simulink model "windModel"  (R2024a)
settings: Solver=VariableStepAuto  StartTime=0.0  StopTime=30  RelTol=1e-3
undefined symbols (not defined in the file or in its folder): F, MIL, Moderate
libraries: aerolibwind2 x2
settings Model: Creator=franklinho  LastModifiedBy=franklinho

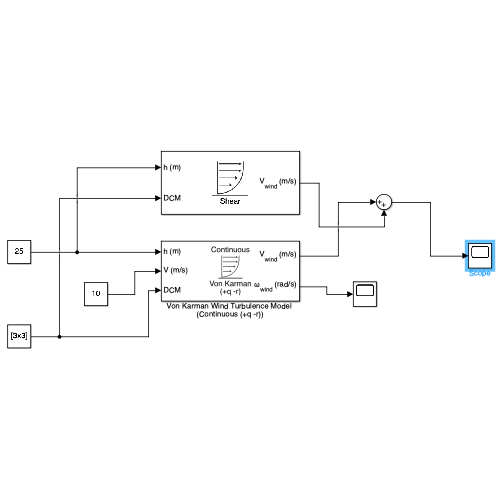
[thumbnail: Simulink's stored preview of the top-level diagram]
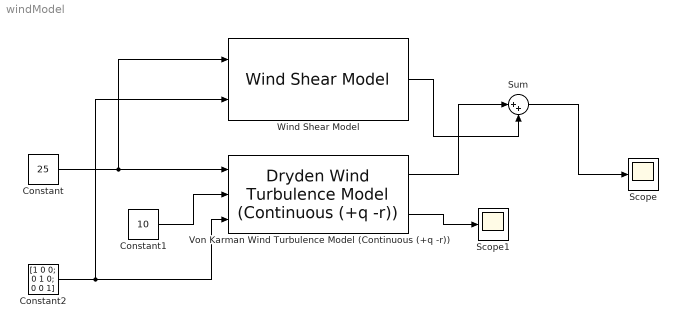
== system windModel ==
  Constant : Constant  Value=25
  Constant1 : Constant  Value=10
  Constant2 : Constant  Value=[1 0 0; 0 1 0; 0 0 1]
  Scope : Scope
  Scope1 : Scope
  Sum : Sum  Inputs=|++
  Von Karman Wind Turbulence Model (Continuous (+q -r)) : aerolibwind2/Dryden Wind Turbulence Model  (Continuous (+q -r))  units=Metric (MKS)  spec=MIL-F-8785C  model=Continuous Von Karman (+q -r)  W20=15  Wdeg=0  TurbProb=10^-3 - Moderate  L_high=762  Wingspan=10  ts=0.001  Seed=[23341 23342 23343 23344]  T_on=on
      settings: LibrarySourceBlock=|
      | aerolibwind2/Von Karman Wind Turbulence Model
      | (Continuous (+q -r))
  Wind Shear Model : aerolibwind2/Wind Shear Model  units=Metric (MKS)  phase=Category C - Terminal Flight Phase  W_20=15  Wdeg=0
  wires:
  Constant1/1 -> Von Karman Wind Turbulence Model (Continuous (+q -r))/2
  Constant2/1 -> Wind Shear Model/2, Von Karman Wind Turbulence Model (Continuous (+q -r))/3
  Constant/1 -> Wind Shear Model/1, Von Karman Wind Turbulence Model (Continuous (+q -r))/1
  Sum/1 -> Scope/1
  Von Karman Wind Turbulence Model (Continuous (+q -r))/2 -> Scope1/1
  Von Karman Wind Turbulence Model (Continuous (+q -r))/1 -> Sum/1
  Wind Shear Model/1 -> Sum/2
